simulink model "TestData"  (R2024a)
settings: Solver=VariableStepAuto  StartTime=0.0  StopTime=15  RelTol=1e-3
libraries: spspowerguiLib x1
settings Model: Creator=fiona  LastModifiedBy=fiona

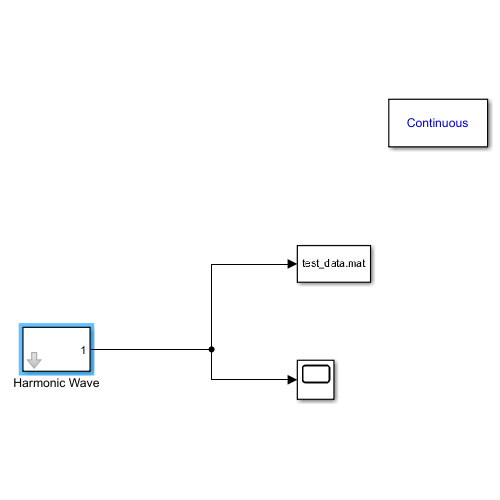
[thumbnail: Simulink's stored preview of the top-level diagram]
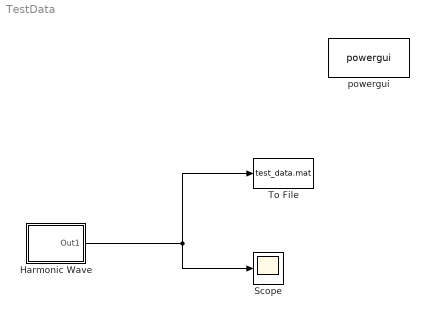
== system TestData ==
  Harmonic Wave : Subsystem  mask{Ampf=16, Amp3=2, Amp5=1, Amp7=0.7, Amp9=0.5, Amp11=0.3, Amp13=0.1}
      mask prompts: Ampf "Fundamental Amplitude:"; Amp3 "3rd Harmonic Amp:"; Amp5 "5th Harmonic Amp:"; Amp7 "7th Harmonic Amp:"; Amp9 "9th Harmonic Amp:"; Amp11 "11th Harmonic Amp:"; Amp13 "13th Harmonic Amp:"
      mask TypeOptions Ampf: Fundamental/Amplitude
      mask TypeOptions Amp3: 3rd Harmonic/Amplitude
      mask TypeOptions Amp5: 5th Harmonic/Amplitude
      mask TypeOptions Amp7: 7th Harmonic/Amplitude
      mask TypeOptions Amp9: 9th Harmonic/Amplitude
      mask TypeOptions Amp11: 11th Harmonic/Amplitude
      mask TypeOptions Amp13: 13th Harmonic/Amplitude
  Scope : Scope
  To File : ToFile  Filename=test_data.mat  MatrixName=field_data
  powergui : spspowerguiLib/powergui  Priority=1  SimulationMode=Continuous  SampleTime=50e-6  frequency=60  Iterations=50  frequencyindice=60  Pbase=100e6  ErrMax=1e-4  UnitsV=kV  UnitsW=MW  buscounter=0  FunctionMessages=off  echomessages=off  EnableUseOfTLC=off  CurrentSourceSwitches=off  DisableSnubberDevices=off  DisableRonSwitches=off  DisableVfSwitches=off  DisplayEquations=off  AutomaticDiscreteSolvers=off  SolverType=Tustin/Backward Euler (TBE)  Interpol=off  ExternalGateDelay=off  methode=off  Ts=100  x0status=blocks  SPID=on  SwTol=0  HookPort=off  NonlinearTolerance=1e-4  nMaxIteration=100  ContinueOnMaxIteration=off  RestoreLinks=warning  ResistiveCurrentMeasurement=off  Frange=[0:2:500]  Ylog=off  Xlog=on  ShowGrid=off  save=off  variable=ZData  structure=0  ZoomFFT=off  StartTime=0.0  cycles=1  DisplayStyle=1  fundamental=60  FreqAxis=off  MaxFrequency=1000  frequencyindicesteady=1  RmsSteady=1  display=off
  wires:
  Harmonic Wave/1(Out1) -> To File/1, Scope/1

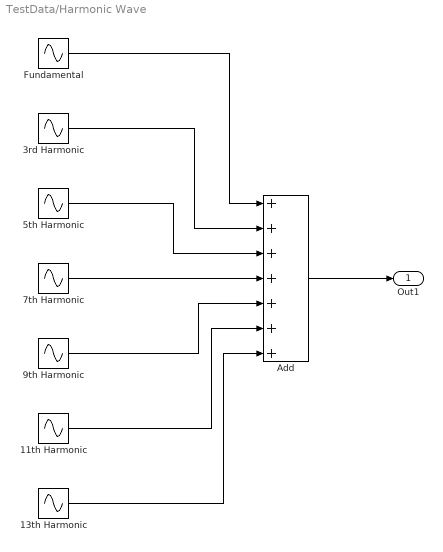
== system TestData/Harmonic Wave ==
  11th Harmonic : Sin  Amplitude=Amp11  Frequency=11*60*(2*pi)  SampleTime=0
  13th Harmonic : Sin  Amplitude=Amp13  Frequency=13*60*(2*pi)  SampleTime=0
  3rd Harmonic : Sin  Amplitude=Amp3  Frequency=3*60*(2*pi)  SampleTime=0
  5th Harmonic : Sin  Amplitude=Amp5  Frequency=5*60*(2*pi)  SampleTime=0
  7th Harmonic : Sin  Amplitude=Amp7  Frequency=7*60*(2*pi)  SampleTime=0
  9th Harmonic : Sin  Amplitude=Amp9  Frequency=9*60*(2*pi)  SampleTime=0
  Add : Sum  Inputs=+++++++
  Fundamental : Sin  Amplitude=Ampf  Frequency=60*(2*pi)  SampleTime=0
  Out1 : Outport
  wires:
  9th Harmonic/1 -> Add/5
  Fundamental/1 -> Add/1
  11th Harmonic/1 -> Add/6
  5th Harmonic/1 -> Add/3
  3rd Harmonic/1 -> Add/2
  7th Harmonic/1 -> Add/4
  13th Harmonic/1 -> Add/7
  Add/1 -> Out1/1
